simulink model "Model_UAV"  (R2024b)
settings: Solver=VariableStepAuto  StartTime=0.0  StopTime=10.0  RelTol=1e-3
values from neighbouring files (symbols this model uses):
  g = 9.81    [main.m]    (also in main2.m; main_with_fixed_t.m; myStepFunction.m; quadrotorStepFunction.m)
  Kd_pos = diag(Action(4:6))    [quadrotorStepFunction.m]
  Kp_pos = diag(Action(1:3))    [quadrotorStepFunction.m]
settings Model: Creator=Alessandro  LastModifiedBy=Alessandro

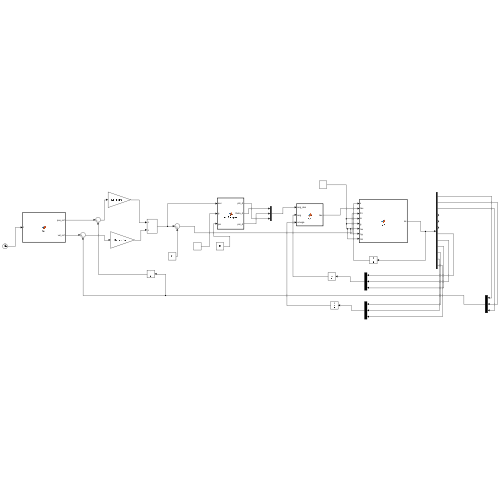
[thumbnail: Simulink's stored preview of the top-level diagram]
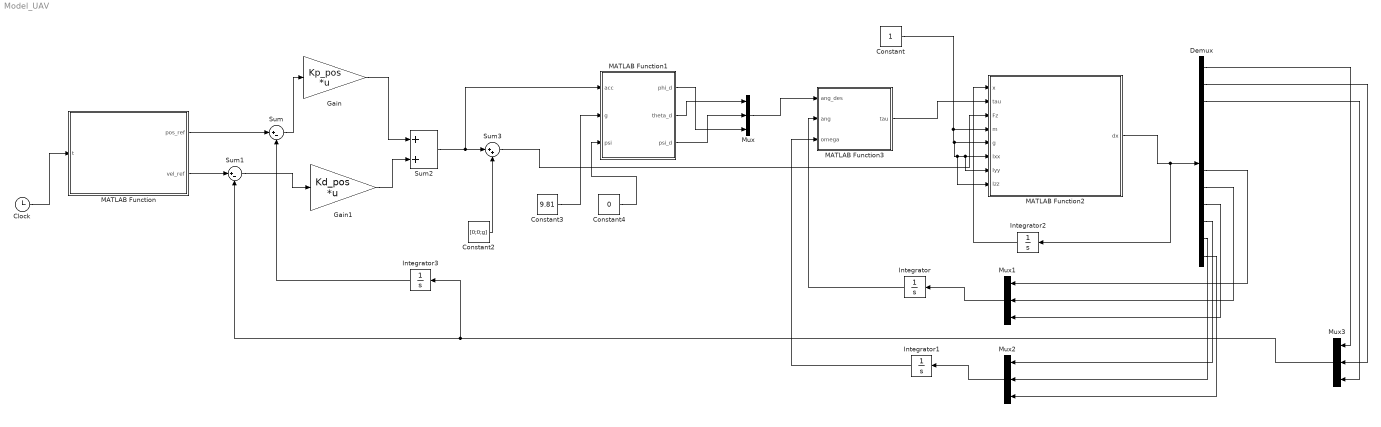
== system Model_UAV ==
  Clock : Clock
  Constant : Constant
  Constant2 : Constant  Value=[0;0;g]
  Constant3 : Constant  Value=9.81
  Constant4 : Constant  Value=0
  Demux : Demux  Outputs=12
  Gain : Gain  Gain=Kp_pos  Multiplication=Matrix(K*u)
  Gain1 : Gain  Gain=Kd_pos  Multiplication=Matrix(K*u)
  Integrator{,1..3} (4 alike) : Integrator
  MATLAB Function : MATLAB Function  TreatAsAtomicUnit=on
  MATLAB Function1 : MATLAB Function  TreatAsAtomicUnit=on
  MATLAB Function2 : MATLAB Function  TreatAsAtomicUnit=on
  MATLAB Function3 : MATLAB Function  TreatAsAtomicUnit=on
  Mux{,1..3} (4 alike) : Mux  Inputs=3
  Sum : Sum  Inputs=|+-
  Sum1 : Sum  Inputs=|+-
  Sum2 : Sum
  Sum3 : Sum  Inputs=|++
  wires:
  Clock/1 -> MATLAB Function/1(t)
  MATLAB Function/1(pos_ref) -> Sum/1
  Sum1/1 -> Gain1/1
  MATLAB Function/2(vel_ref) -> Sum1/1
  Sum/1 -> Gain/1
  Gain/1 -> Sum2/1
  Gain1/1 -> Sum2/2
  Sum2/1 -> MATLAB Function1/1(acc), Sum3/1
  Constant2/1 -> Sum3/2
  Constant3/1 -> MATLAB Function1/2(g)
  Constant4/1 -> MATLAB Function1/3(psi)
  MATLAB Function3/1(tau) -> MATLAB Function2/2(tau)
  MATLAB Function1/1(phi_d) -> Mux/3
  MATLAB Function1/2(theta_d) -> Mux/1
  MATLAB Function1/3(psi_d) -> Mux/2
  Mux/1 -> MATLAB Function3/1(ang_des)
  MATLAB Function2/1(dx) -> Integrator2/1, Demux/1
  Demux/7 -> Mux1/1
  Demux/8 -> Mux1/2
  Demux/9 -> Mux1/3
  Integrator/1 -> MATLAB Function3/2(ang)
  Mux1/1 -> Integrator/1
  Mux2/1 -> Integrator1/1
  Integrator1/1 -> MATLAB Function3/3(omega)
  Demux/10 -> Mux2/1
  Demux/11 -> Mux2/2
  Demux/12 -> Mux2/3
  Integrator2/1 -> MATLAB Function2/1(x)
  Demux/1 -> Mux3/1
  Demux/2 -> Mux3/2
  Demux/3 -> Mux3/3
  Mux3/1 -> Integrator3/1, Sum1/2
  Integrator3/1 -> Sum/2
  Sum3/1 -> MATLAB Function2/3(Fz)
  Constant/1 -> MATLAB Function2/8(Izz), MATLAB Function2/7(Iyy), MATLAB Function2/6(Ixx), MATLAB Function2/5(g), MATLAB Function2/4(m)

== matlab function Model_UAV/MATLAB Function1 ==
  data: acc input; phi_d output; g input; psi input; theta_d output; psi_d output
function [phi_d, theta_d, psi_d] = acc2angles(acc, g, psi)
    phi_d = (1/g)*(acc(1)*sin(psi) - acc(2)*cos(psi));
    theta_d = (1/g)*(acc(1)*cos(psi) + acc(2)*sin(psi));
    psi_d = 0;  % fissa
end

== matlab function Model_UAV/MATLAB Function ==
  data: t input; pos_ref output; vel_ref output
function [pos_ref, vel_ref] = fcn(t)
    if t < 5
        pos_ref = [2*t/5; 0; 2];
        vel_ref = [2/5; 0; 0];
    elseif t < 10
        pos_ref = [2; 2*(t-5)/5; 2];
        vel_ref = [0; 2/5; 0];
    else
        pos_ref = [2 - 2*(t-10)/5; 2; 2];
        vel_ref = [-2/5; 0; 0];
    end
end

== matlab function Model_UAV/MATLAB Function2 ==
  data: x input; dx output size=12; tau input; Fz input; m input; g input; Ixx input; Iyy input; Izz input
function dx = fcn(x, tau, Fz, m, g, Ixx, Iyy, Izz)
    pos = x(1:3); vel = x(4:6);
    phi = x(7); theta = x(8); psi = x(9);
    omega = x(10:12);

    % Rotazione
    R = eul2rotm([psi, theta, phi]);
    acc = (1/m)*(R * [0; 0; Fz]) - [0; 0; g];

    omega_dot = [ ...
        (tau(1) - (Iyy - Izz)*omega(2)*omega(3)) / Ixx;
        (tau(2) - (Izz - Ixx)*omega(1)*omega(3)) / Iyy;
        (tau(3) - (Ixx - Iyy)*omega(1)*omega(2)) / Izz ];

    % Derivate angoli
    phi_dot = omega(1) + tan(theta)*(omega(2)*sin(phi) + omega(3)*cos(phi));
    theta_dot = omega(2)*cos(phi) - omega(3)*sin(phi);
    psi_dot = (omega(2)*sin(phi) + omega(3)*cos(phi))/cos(theta);

    dx = zeros(12,1);
    dx(1:3) = vel;
    dx(4:6) = acc;
    dx(7) = phi_dot;
    dx(8) = theta_dot;
    dx(9) = psi_dot;
    dx(10:12) = omega_dot;
end

function R = eul2rotm(eul)
    psi = eul(1); theta = eul(2); phi = eul(3);
    Rz = [cos(psi) -sin(psi) 0; sin(psi) cos(psi) 0; 0 0 1];
    Ry = [cos(theta) 0 sin(theta); 0 1 0; -sin(theta) 0 cos(theta)];
    Rx = [1 0 0; 0 cos(phi) -sin(phi); 0 sin(phi) cos(phi)];
    R = Rz * Ry * Rx;
end

== matlab function Model_UAV/MATLAB Function3 ==
  data: ang_des input; tau output; ang input; omega input
function tau = fcn(ang_des, ang, omega)
    Kp_ang = diag([150, 150, 100]);
    Kd_ang = diag([50, 50, 30]);

    e_ang = ang_des - ang;
    e_omega = -omega;

    tau = Kp_ang * e_ang + Kd_ang * e_omega;
end
